simulink model "v_blast_t4_r4"  (Simulink 6.1)
settings: Solver=ode45  StartTime=0.0  StopTime=1.25  RelTol=1e-3
values from neighbouring files (symbols this model uses):
  Tsym = 1.25e-6    (= 1.25e-06)    [initial.m]
libraries: commchan2 x20, simulink x16, dspmtrx3 x14, dspbuff3 x6, dspinverses x2, commdigbbndpm2 x2, commsink2 x1, dspobslib x1, dspindex x1, commrandsrc2 x1
settings Model: LastModifiedBy=ncl2
settings DebuggingCC: SolverPrmCheckMsg=warning

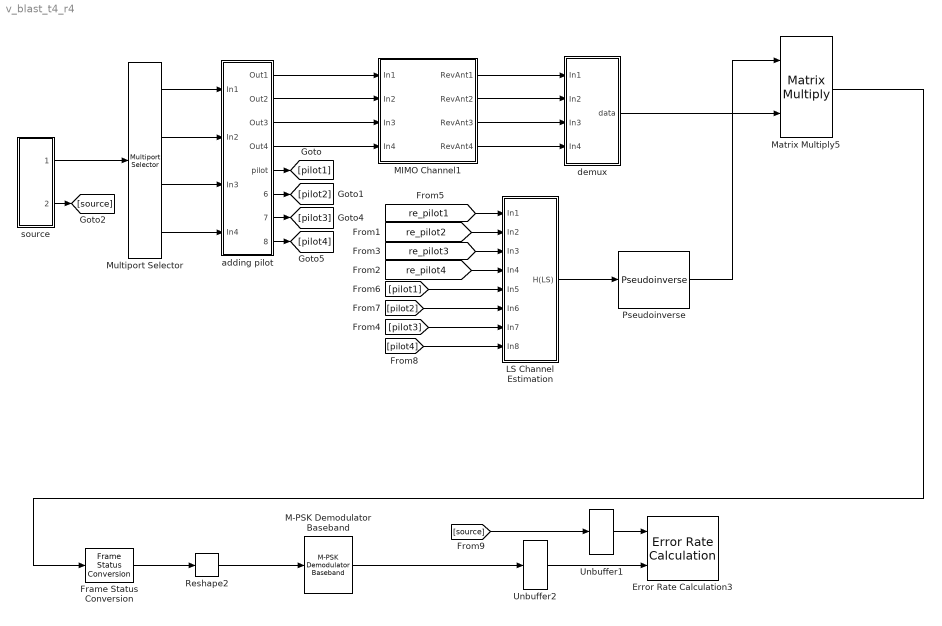
== system v_blast_t4_r4 ==
  Error Rate Calculation3 : commsink2/Error Rate Calculation  N=256*3  st_delay=0  cp_mode=Entire frame  subframe=[]  PMode=Workspace  WsName=Error  RsMode2=off  stop=off  numErr=3e5  maxBits=3e5
  Frame Status Conversion : dspobslib/Frame Status Conversion  growRefPort=off  outframe=Frame-based
  LS Channel Estimation : Subsystem
  M-PSK Demodulator Baseband : commdigbbndpm2/M-PSK Demodulator Baseband  M=8  OutType=Bit  Dec=Binary  Ph=0  numSamp=1
  MIMO Channel1 : Subsystem
  Matrix Multiply5 : dspmtrx3/Matrix Multiply  numInputPorts=2  OptimizationLevel=None
  Multiport Selector : dspindex/Multiport Selector  Tag=S/P  Description=S/P  rowsOrCols=Rows  idxCellArray={1,2,3,4}  idxErrMode=Clip Index
  Pseudoinverse : dspinverses/Pseudoinverse
  Reshape2 : simulink/Math Operations/Reshape  OutputDimensionality=Column vector  OutputDimensions=[1,1]
  Unbuffer1 : dspbuff3/Unbuffer  ic=0
  Unbuffer2 : dspbuff3/Unbuffer  ic=0
  adding pilot : Subsystem
  demux : Subsystem
  source : Subsystem
  wires:
  Unbuffer1/1 -> Error Rate Calculation3/1
  Unbuffer2/1 -> Error Rate Calculation3/2
  source/2(Out2) -> [source]
  [source] -> Unbuffer1/1
  [pilot4] -> LS Channel Estimation/8(In8)
  [pilot3] -> LS Channel Estimation/7(In7)
  [re_pilot4] -> LS Channel Estimation/4(In4)
  [re_pilot3] -> LS Channel Estimation/3(In3)
  MIMO Channel1/4(RevAnt4) -> demux/4(In4)
  MIMO Channel1/3(RevAnt3) -> demux/3(In3)
  MIMO Channel1/2(RevAnt2) -> demux/2(In2)
  MIMO Channel1/1(RevAnt1) -> demux/1(In1)
  adding pilot/4(Out4) -> MIMO Channel1/4(In4)
  adding pilot/3(Out3) -> MIMO Channel1/3(In3)
  adding pilot/2(Out2) -> MIMO Channel1/2(In2)
  adding pilot/1(Out1) -> MIMO Channel1/1(In1)
  adding pilot/8(pilot3) -> [pilot4]
  adding pilot/7(pilot2) -> [pilot3]
  Multiport Selector/4 -> adding pilot/4(In4)
  Multiport Selector/3 -> adding pilot/3(In3)
  Reshape2/1 -> M-PSK Demodulator Baseband/1
  LS Channel Estimation/1(H(LS)) -> Pseudoinverse/1
  [pilot2] -> LS Channel Estimation/6(In6)
  [pilot1] -> LS Channel Estimation/5(In5)
  [re_pilot2] -> LS Channel Estimation/2(In2)
  [re_pilot1] -> LS Channel Estimation/1(In1)
  adding pilot/6(pilot1) -> [pilot2]
  adding pilot/5(pilot) -> [pilot1]
  Multiport Selector/2 -> adding pilot/2(In2)
  Multiport Selector/1 -> adding pilot/1(In1)
  Frame Status Conversion/1 -> Reshape2/1
  Matrix Multiply5/1 -> Frame Status Conversion/1
  M-PSK Demodulator Baseband/1 -> Unbuffer2/1
  demux/1(data) -> Matrix Multiply5/2
  Pseudoinverse/1 -> Matrix Multiply5/1
  source/1(Out1) -> Multiport Selector/1

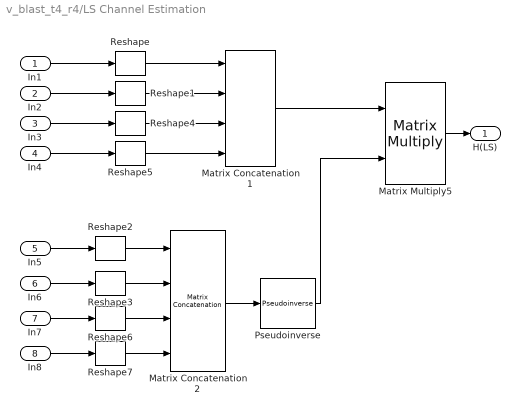
== system v_blast_t4_r4/LS Channel Estimation ==
  In1 : Inport  Port=1  LatchInput=off
  In2 : Inport  Port=2  LatchInput=off
  In3 : Inport  Port=3  LatchInput=off
  In4 : Inport  Port=4  LatchInput=off
  In5 : Inport  Port=5  LatchInput=off
  In6 : Inport  Port=6  LatchInput=off
  In7 : Inport  Port=7  LatchInput=off
  In8 : Inport  Port=8  LatchInput=off
  Matrix Concatenation1 : simulink/Math Operations/Matrix Concatenation  numInports=4  catMethod=Vertical
  Matrix Concatenation2 : simulink/Math Operations/Matrix Concatenation  numInports=4  catMethod=Vertical
  Matrix Multiply5 : dspmtrx3/Matrix Multiply  numInputPorts=2  OptimizationLevel=None
  Pseudoinverse : dspinverses/Pseudoinverse
  Reshape{,1..7} (8 alike) : simulink/Math Operations/Reshape  OutputDimensionality=Row vector  OutputDimensions=[1,1]
  H(LS) : Outport
  wires:
  Reshape/1 -> Matrix Concatenation1/1
  Reshape1/1 -> Matrix Concatenation1/2
  In1/1 -> Reshape/1
  Matrix Concatenation1/1 -> Matrix Multiply5/1
  In2/1 -> Reshape1/1
  Reshape2/1 -> Matrix Concatenation2/1
  Reshape3/1 -> Matrix Concatenation2/2
  In5/1 -> Reshape2/1
  Matrix Concatenation2/1 -> Pseudoinverse/1
  In6/1 -> Reshape3/1
  Pseudoinverse/1 -> Matrix Multiply5/2
  Matrix Multiply5/1 -> H(LS)/1
  In3/1 -> Reshape4/1
  In4/1 -> Reshape5/1
  Reshape4/1 -> Matrix Concatenation1/3
  Reshape5/1 -> Matrix Concatenation1/4
  In7/1 -> Reshape6/1
  In8/1 -> Reshape7/1
  Reshape6/1 -> Matrix Concatenation2/3
  Reshape7/1 -> Matrix Concatenation2/4

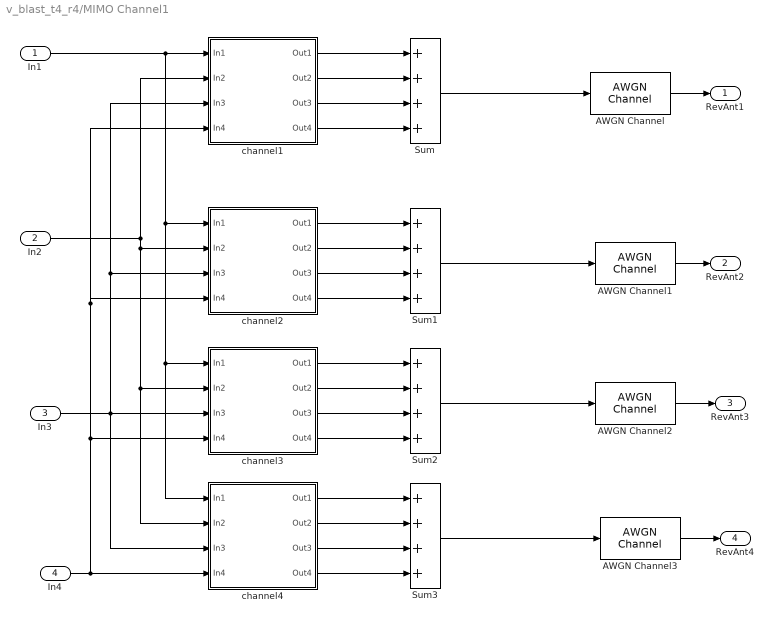
== system v_blast_t4_r4/MIMO Channel1 ==
  In1 : Inport  Port=1  LatchInput=off
  In2 : Inport  Port=2  LatchInput=off
  In3 : Inport  Port=3  LatchInput=off
  In4 : Inport  Port=4  LatchInput=off
  AWGN Channel : commchan2/AWGN Channel  seed=167  noiseMode="Signal to noise ratio  (Eb/No)"  EbNodB=SNR  EsNodB=10  SNRdB=Snr  bitsPerSym=3  Ps=Ps  Tsym=3*Tsym  variance=1
  AWGN Channel1 : commchan2/AWGN Channel  seed=16712  noiseMode="Signal to noise ratio  (Eb/No)"  EbNodB=SNR  EsNodB=10  SNRdB=Snr  bitsPerSym=3  Ps=Ps  Tsym=3*Tsym  variance=1
  AWGN Channel2 : commchan2/AWGN Channel  seed=367  noiseMode="Signal to noise ratio  (Eb/No)"  EbNodB=SNR  EsNodB=10  SNRdB=Snr  bitsPerSym=3  Ps=Ps  Tsym=3*Tsym  variance=1
  AWGN Channel3 : commchan2/AWGN Channel  seed=4671  noiseMode="Signal to noise ratio  (Eb/No)"  EbNodB=SNR  EsNodB=10  SNRdB=Snr  bitsPerSym=3  Ps=Ps  Tsym=3*Tsym  variance=1
  Sum{,1..3} (4 alike) : Sum  Inputs=++++  SaturateOnIntegerOverflow=on
  channel1 : Subsystem
  channel2 : Subsystem
  channel3 : Subsystem
  channel4 : Subsystem
  RevAnt1 : Outport
  RevAnt2 : Outport  Port=2
  RevAnt3 : Outport  Port=3
  RevAnt4 : Outport  Port=4
  wires:
  channel1/2(Out2) -> Sum/2
  channel1/1(Out1) -> Sum/1
  Sum/1 -> AWGN Channel/1
  Sum1/1 -> AWGN Channel1/1
  In1/1 -> channel1/1(In1), channel3/1(In1), channel4/1(In1), channel2/1(In1)
  In2/1 -> channel1/2(In2), channel2/2(In2), channel3/2(In2), channel4/2(In2)
  AWGN Channel/1 -> RevAnt1/1
  AWGN Channel1/1 -> RevAnt2/1
  channel2/1(Out1) -> Sum1/1
  channel2/2(Out2) -> Sum1/2
  channel2/3(Out3) -> Sum1/3
  channel2/4(Out4) -> Sum1/4
  channel3/1(Out1) -> Sum2/1
  channel3/2(Out2) -> Sum2/2
  channel3/3(Out3) -> Sum2/3
  channel3/4(Out4) -> Sum2/4
  channel4/1(Out1) -> Sum3/1
  channel4/2(Out2) -> Sum3/2
  channel4/3(Out3) -> Sum3/3
  channel4/4(Out4) -> Sum3/4
  AWGN Channel2/1 -> RevAnt3/1
  AWGN Channel3/1 -> RevAnt4/1
  Sum3/1 -> AWGN Channel3/1
  Sum2/1 -> AWGN Channel2/1
  In3/1 -> channel3/3(In3), channel1/3(In3), channel2/3(In3), channel4/3(In3)
  In4/1 -> channel4/4(In4), channel3/4(In4), channel2/4(In4), channel1/4(In4)
  channel1/3(Out3) -> Sum/3
  channel1/4(Out4) -> Sum/4

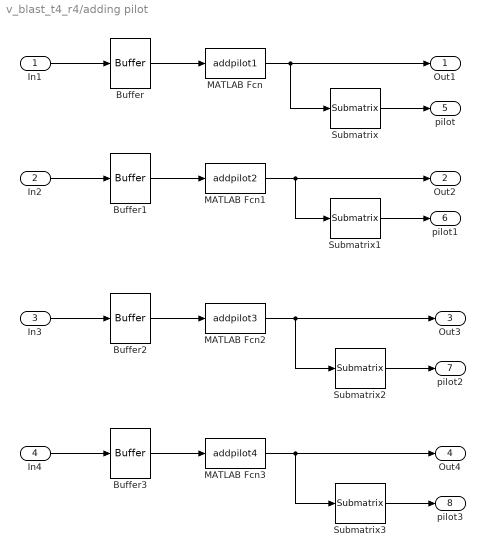
== system v_blast_t4_r4/adding pilot ==
  In1 : Inport  Port=1  LatchInput=off
  In2 : Inport  Port=2  LatchInput=off
  In3 : Inport  Port=3  LatchInput=off
  In4 : Inport  Port=4  LatchInput=off
  Buffer{,1..3} (4 alike) : dspbuff3/Buffer  N=256  V=0  ic=0
  MATLAB Fcn : MATLABFcn  MATLABFcn=addpilot1  Output1D=off
  MATLAB Fcn1 : MATLABFcn  MATLABFcn=addpilot2  Output1D=off
  MATLAB Fcn2 : MATLABFcn  MATLABFcn=addpilot3  Output1D=off
  MATLAB Fcn3 : MATLABFcn  MATLABFcn=addpilot4  Output1D=off
  Submatrix{,1..3} (4 alike) : dspmtrx3/Submatrix  RowSpan=Range of rows  RowStartMode=Index  RowStartIndex=256+1  RowEndMode=Index  RowEndIndex=256+64  ColSpan=Range of columns  ColStartMode=First  ColStartIndex=1  ColEndMode=Last  ColEndIndex=1
  Out1 : Outport
  Out2 : Outport  Port=2
  Out3 : Outport  Port=3
  Out4 : Outport  Port=4
  pilot : Outport  Port=5
  pilot1 : Outport  Port=6
  pilot2 : Outport  Port=7
  pilot3 : Outport  Port=8
  wires:
  In1/1 -> Buffer/1
  In2/1 -> Buffer1/1
  Submatrix/1 -> pilot/1
  In3/1 -> Buffer2/1
  In4/1 -> Buffer3/1
  Buffer3/1 -> MATLAB Fcn3/1
  Buffer2/1 -> MATLAB Fcn2/1
  Buffer1/1 -> MATLAB Fcn1/1
  Buffer/1 -> MATLAB Fcn/1
  MATLAB Fcn1/1 -> Out2/1, Submatrix1/1
  Submatrix1/1 -> pilot1/1
  MATLAB Fcn2/1 -> Submatrix2/1, Out3/1
  Submatrix2/1 -> pilot2/1
  MATLAB Fcn3/1 -> Out4/1, Submatrix3/1
  Submatrix3/1 -> pilot3/1
  MATLAB Fcn/1 -> Out1/1, Submatrix/1

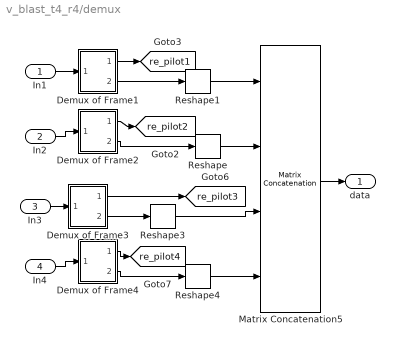
== system v_blast_t4_r4/demux ==
  In1 : Inport  Port=1  LatchInput=off
  In2 : Inport  Port=2  LatchInput=off
  In3 : Inport  Port=3  LatchInput=off
  In4 : Inport  Port=4  LatchInput=off
  Demux of Frame1 : Subsystem
  Demux of Frame2 : Subsystem
  Demux of Frame3 : Subsystem
  Demux of Frame4 : Subsystem
  Matrix Concatenation5 : simulink/Math Operations/Matrix Concatenation  numInports=4  catMethod=Vertical
  Reshape{,1,3..4} (4 alike) : simulink/Math Operations/Reshape  OutputDimensionality=Row vector  OutputDimensions=[1,1]
  data : Outport
  tag scope: re_pilot1=global, re_pilot2=global, re_pilot3=global, re_pilot4=global
  wires:
  Demux of Frame2/2(Out3) -> Reshape/1
  Demux of Frame2/1(Out1) -> [re_pilot2]
  Demux of Frame1/1(Out1) -> [re_pilot1]
  Demux of Frame1/2(Out3) -> Reshape1/1
  Demux of Frame3/2(Out3) -> Reshape3/1
  Demux of Frame3/1(Out1) -> [re_pilot3]
  Demux of Frame4/1(Out1) -> [re_pilot4]
  Demux of Frame4/2(Out3) -> Reshape4/1
  Reshape1/1 -> Matrix Concatenation5/1
  Reshape/1 -> Matrix Concatenation5/2
  Reshape3/1 -> Matrix Concatenation5/3
  Reshape4/1 -> Matrix Concatenation5/4
  In1/1 -> Demux of Frame1/1(In1)
  In2/1 -> Demux of Frame2/1(In1)
  Matrix Concatenation5/1 -> data/1
  In3/1 -> Demux of Frame3/1(In1)
  In4/1 -> Demux of Frame4/1(In1)

== system v_blast_t4_r4/source ==
  Bernoulli Binary Generator : commrandsrc2/Bernoulli Binary Generator  P=0.5  seed=61  Ts=Tsym  frameBased=on  sampPerFrame=3  orient=off
  M-PSK Modulator Baseband : commdigbbndpm2/M-PSK Modulator Baseband  M=8  InType=Bit  Enc=Binary  Ph=0  numSamp=1
  Out1 : Outport
  Out2 : Outport  Orientation=left  Port=2
  wires:
  Bernoulli Binary Generator/1 -> Out2/1, M-PSK Modulator Baseband/1
  M-PSK Modulator Baseband/1 -> Out1/1

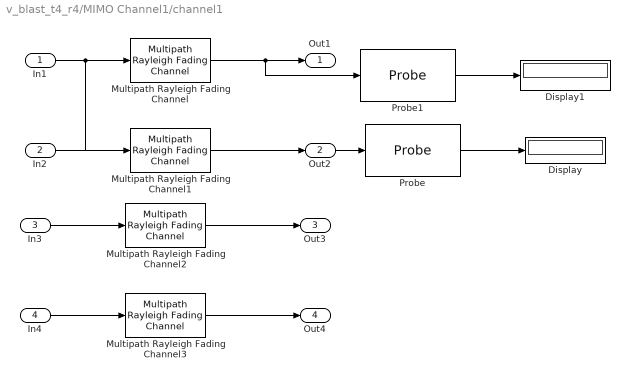
== system v_blast_t4_r4/MIMO Channel1/channel1 ==
  In1 : Inport  Port=1  LatchInput=off
  In2 : Inport  Port=2  LatchInput=off
  In3 : Inport  Port=3  LatchInput=off
  In4 : Inport  Port=4  LatchInput=off
  Display : Display
  Display1 : Display
  Multipath Rayleigh Fading Channel : commchan2/Multipath Rayleigh Fading Channel  Fd=Fdmax  simTs=SampleTime  delayVec=0  gainVecdB=0  normGain=on  Seed=1234
  Multipath Rayleigh Fading Channel1 : commchan2/Multipath Rayleigh Fading Channel  Fd=Fdmax  simTs=SampleTime  delayVec=0  gainVecdB=0  normGain=on  Seed=2345
  Multipath Rayleigh Fading Channel2 : commchan2/Multipath Rayleigh Fading Channel  Fd=Fdmax  simTs=SampleTime  delayVec=0  gainVecdB=0  normGain=on  Seed=4567
  Multipath Rayleigh Fading Channel3 : commchan2/Multipath Rayleigh Fading Channel  Fd=Fdmax  simTs=SampleTime  delayVec=0  gainVecdB=0  normGain=on  Seed=6789
  Probe : Probe  ProbeWidth=off  ProbeComplexSignal=off
  Probe1 : Probe  ProbeWidth=off  ProbeComplexSignal=off
  Out1 : Outport
  Out2 : Outport  Port=2
  Out3 : Outport  Port=3
  Out4 : Outport  Port=4
  wires:
  In1/1 -> Multipath Rayleigh Fading Channel/1, Probe/1
  In2/1 -> Multipath Rayleigh Fading Channel1/1
  Multipath Rayleigh Fading Channel/1 -> Out1/1, Probe1/1
  Multipath Rayleigh Fading Channel1/1 -> Out2/1
  In3/1 -> Multipath Rayleigh Fading Channel2/1
  In4/1 -> Multipath Rayleigh Fading Channel3/1
  Multipath Rayleigh Fading Channel2/1 -> Out3/1
  Multipath Rayleigh Fading Channel3/1 -> Out4/1
  Probe/1 -> Display/1
  Probe1/1 -> Display1/1

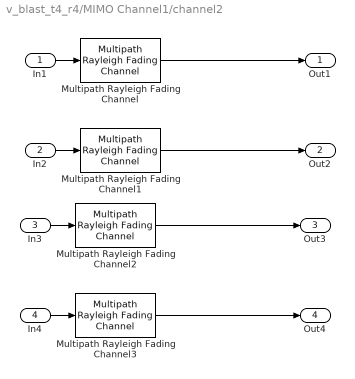
== system v_blast_t4_r4/MIMO Channel1/channel2 ==
  In1 : Inport  Port=1  LatchInput=off
  In2 : Inport  Port=2  LatchInput=off
  In3 : Inport  Port=3  LatchInput=off
  In4 : Inport  Port=4  LatchInput=off
  Multipath Rayleigh Fading Channel : commchan2/Multipath Rayleigh Fading Channel  Fd=Fdmax  simTs=SampleTime  delayVec=0  gainVecdB=0  normGain=on  Seed=1345
  Multipath Rayleigh Fading Channel1 : commchan2/Multipath Rayleigh Fading Channel  Fd=Fdmax  simTs=SampleTime  delayVec=0  gainVecdB=0  normGain=on  Seed=2456
  Multipath Rayleigh Fading Channel2 : commchan2/Multipath Rayleigh Fading Channel  Fd=Fdmax  simTs=SampleTime  delayVec=0  gainVecdB=0  normGain=on  Seed=3567
  Multipath Rayleigh Fading Channel3 : commchan2/Multipath Rayleigh Fading Channel  Fd=Fdmax  simTs=SampleTime  delayVec=0  gainVecdB=0  normGain=on  Seed=4678
  Out1 : Outport
  Out2 : Outport  Port=2
  Out3 : Outport  Port=3
  Out4 : Outport  Port=4
  wires:
  Multipath Rayleigh Fading Channel3/1 -> Out4/1
  Multipath Rayleigh Fading Channel2/1 -> Out3/1
  In4/1 -> Multipath Rayleigh Fading Channel3/1
  In3/1 -> Multipath Rayleigh Fading Channel2/1
  Multipath Rayleigh Fading Channel1/1 -> Out2/1
  Multipath Rayleigh Fading Channel/1 -> Out1/1
  In2/1 -> Multipath Rayleigh Fading Channel1/1
  In1/1 -> Multipath Rayleigh Fading Channel/1

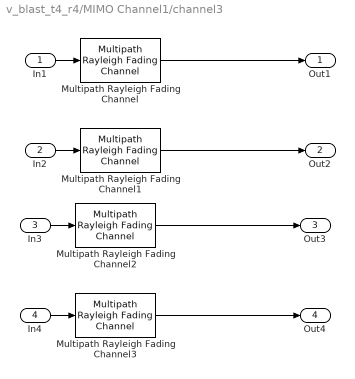
== system v_blast_t4_r4/MIMO Channel1/channel3 ==
  In1 : Inport  Port=1  LatchInput=off
  In2 : Inport  Port=2  LatchInput=off
  In3 : Inport  Port=3  LatchInput=off
  In4 : Inport  Port=4  LatchInput=off
  Multipath Rayleigh Fading Channel : commchan2/Multipath Rayleigh Fading Channel  Fd=Fdmax  simTs=SampleTime  delayVec=0  gainVecdB=0  normGain=on  Seed=2567
  Multipath Rayleigh Fading Channel1 : commchan2/Multipath Rayleigh Fading Channel  Fd=Fdmax  simTs=SampleTime  delayVec=0  gainVecdB=0  normGain=on  Seed=3678
  Multipath Rayleigh Fading Channel2 : commchan2/Multipath Rayleigh Fading Channel  Fd=Fdmax  simTs=SampleTime  delayVec=0  gainVecdB=0  normGain=on  Seed=4789
  Multipath Rayleigh Fading Channel3 : commchan2/Multipath Rayleigh Fading Channel  Fd=Fdmax  simTs=SampleTime  delayVec=0  gainVecdB=0  normGain=on  Seed=5432
  Out1 : Outport
  Out2 : Outport  Port=2
  Out3 : Outport  Port=3
  Out4 : Outport  Port=4
  wires:
  In1/1 -> Multipath Rayleigh Fading Channel/1
  In2/1 -> Multipath Rayleigh Fading Channel1/1
  Multipath Rayleigh Fading Channel/1 -> Out1/1
  Multipath Rayleigh Fading Channel1/1 -> Out2/1
  In3/1 -> Multipath Rayleigh Fading Channel2/1
  In4/1 -> Multipath Rayleigh Fading Channel3/1
  Multipath Rayleigh Fading Channel2/1 -> Out3/1
  Multipath Rayleigh Fading Channel3/1 -> Out4/1

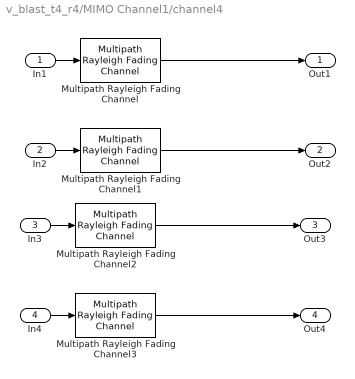
== system v_blast_t4_r4/MIMO Channel1/channel4 ==
  In1 : Inport  Port=1  LatchInput=off
  In2 : Inport  Port=2  LatchInput=off
  In3 : Inport  Port=3  LatchInput=off
  In4 : Inport  Port=4  LatchInput=off
  Multipath Rayleigh Fading Channel : commchan2/Multipath Rayleigh Fading Channel  Fd=Fdmax  simTs=SampleTime  delayVec=0  gainVecdB=0  normGain=on  Seed=4321
  Multipath Rayleigh Fading Channel1 : commchan2/Multipath Rayleigh Fading Channel  Fd=Fdmax  simTs=SampleTime  delayVec=0  gainVecdB=0  normGain=on  Seed=9876
  Multipath Rayleigh Fading Channel2 : commchan2/Multipath Rayleigh Fading Channel  Fd=Fdmax  simTs=SampleTime  delayVec=0  gainVecdB=0  normGain=on  Seed=6543
  Multipath Rayleigh Fading Channel3 : commchan2/Multipath Rayleigh Fading Channel  Fd=Fdmax  simTs=SampleTime  delayVec=0  gainVecdB=0  normGain=on  Seed=1456
  Out1 : Outport
  Out2 : Outport  Port=2
  Out3 : Outport  Port=3
  Out4 : Outport  Port=4
  wires:
  Multipath Rayleigh Fading Channel3/1 -> Out4/1
  Multipath Rayleigh Fading Channel2/1 -> Out3/1
  In4/1 -> Multipath Rayleigh Fading Channel3/1
  In3/1 -> Multipath Rayleigh Fading Channel2/1
  Multipath Rayleigh Fading Channel1/1 -> Out2/1
  Multipath Rayleigh Fading Channel/1 -> Out1/1
  In2/1 -> Multipath Rayleigh Fading Channel1/1
  In1/1 -> Multipath Rayleigh Fading Channel/1

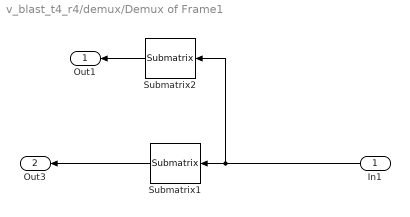
== system v_blast_t4_r4/demux/Demux of Frame1 ==
  In1 : Inport  Orientation=left  Port=1  LatchInput=off
  Submatrix1 : dspmtrx3/Submatrix  Orientation=left  RowSpan=Range of rows  RowStartMode=Index  RowStartIndex=1  RowEndMode=Index  RowEndIndex=256  ColSpan=All columns  ColStartMode=First  ColStartIndex=1  ColEndMode=Last  ColEndIndex=1
  Submatrix2 : dspmtrx3/Submatrix  Orientation=left  RowSpan=Range of rows  RowStartMode=Index  RowStartIndex=256+1  RowEndMode=Index  RowEndIndex=256+64  ColSpan=All columns  ColStartMode=First  ColStartIndex=1  ColEndMode=Last  ColEndIndex=1
  Out1 : Outport  Orientation=left
  Out3 : Outport  Orientation=left  Port=2
  wires:
  Submatrix2/1 -> Out1/1
  Submatrix1/1 -> Out3/1
  In1/1 -> Submatrix2/1, Submatrix1/1

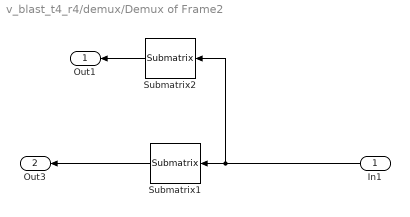
== system v_blast_t4_r4/demux/Demux of Frame2 ==
  In1 : Inport  Orientation=left  Port=1  LatchInput=off
  Submatrix1 : dspmtrx3/Submatrix  Orientation=left  RowSpan=Range of rows  RowStartMode=Index  RowStartIndex=1  RowEndMode=Index  RowEndIndex=256  ColSpan=All columns  ColStartMode=First  ColStartIndex=1  ColEndMode=Last  ColEndIndex=1
  Submatrix2 : dspmtrx3/Submatrix  Orientation=left  RowSpan=Range of rows  RowStartMode=Index  RowStartIndex=256+1  RowEndMode=Index  RowEndIndex=256+64  ColSpan=All columns  ColStartMode=First  ColStartIndex=1  ColEndMode=Last  ColEndIndex=1
  Out1 : Outport  Orientation=left
  Out3 : Outport  Orientation=left  Port=2
  wires:
  In1/1 -> Submatrix1/1, Submatrix2/1
  Submatrix1/1 -> Out3/1
  Submatrix2/1 -> Out1/1

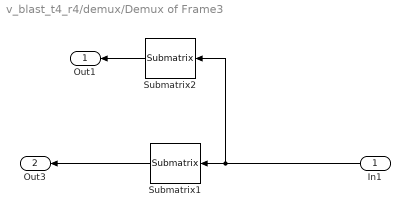
== system v_blast_t4_r4/demux/Demux of Frame3 ==
  In1 : Inport  Orientation=left  Port=1  LatchInput=off
  Submatrix1 : dspmtrx3/Submatrix  Orientation=left  RowSpan=Range of rows  RowStartMode=Index  RowStartIndex=1  RowEndMode=Index  RowEndIndex=256  ColSpan=All columns  ColStartMode=First  ColStartIndex=1  ColEndMode=Last  ColEndIndex=1
  Submatrix2 : dspmtrx3/Submatrix  Orientation=left  RowSpan=Range of rows  RowStartMode=Index  RowStartIndex=256+1  RowEndMode=Index  RowEndIndex=256+64  ColSpan=All columns  ColStartMode=First  ColStartIndex=1  ColEndMode=Last  ColEndIndex=1
  Out1 : Outport  Orientation=left
  Out3 : Outport  Orientation=left  Port=2
  wires:
  Submatrix2/1 -> Out1/1
  Submatrix1/1 -> Out3/1
  In1/1 -> Submatrix2/1, Submatrix1/1

== system v_blast_t4_r4/demux/Demux of Frame4 ==
  In1 : Inport  Orientation=left  Port=1  LatchInput=off
  Submatrix1 : dspmtrx3/Submatrix  Orientation=left  RowSpan=Range of rows  RowStartMode=Index  RowStartIndex=1  RowEndMode=Index  RowEndIndex=256  ColSpan=All columns  ColStartMode=First  ColStartIndex=1  ColEndMode=Last  ColEndIndex=1
  Submatrix2 : dspmtrx3/Submatrix  Orientation=left  RowSpan=Range of rows  RowStartMode=Index  RowStartIndex=256+1  RowEndMode=Index  RowEndIndex=256+64  ColSpan=All columns  ColStartMode=First  ColStartIndex=1  ColEndMode=Last  ColEndIndex=1
  Out1 : Outport  Orientation=left
  Out3 : Outport  Orientation=left  Port=2
  wires:
  In1/1 -> Submatrix1/1, Submatrix2/1
  Submatrix1/1 -> Out3/1
  Submatrix2/1 -> Out1/1
